simulink model "Communication2_2018a"  (R2018a)
settings: Solver=VariableStepAuto  StartTime=0.0  StopTime=0.6  RelTol=1e-3
settings Model: Creator=86188  LastModifiedBy=bzhan

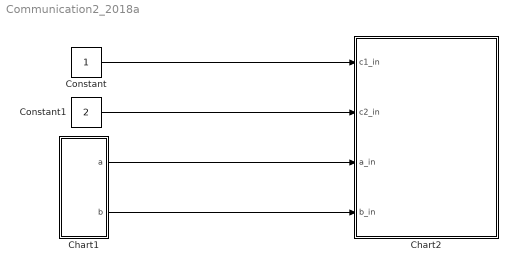
== system Communication2_2018a ==
  Chart1 : Stateflow chart  TreatAsAtomicUnit=on
  Chart2 : Stateflow chart  TreatAsAtomicUnit=on
  Constant : Constant
  Constant1 : Constant  Value=2
  wires:
  Constant1/1 -> Chart2/2(c2_in)
  Constant/1 -> Chart2/1(c1_in)
  Chart1/1(a) -> Chart2/3(a_in)
  Chart1/2(b) -> Chart2/4(b_in)

== stateflow chart Communication2_2018a/Chart2 ==
  settings: updateMethod=DISCRETE  sampleTime=0.1
  state A1
    en: g("en_A1");
    du: f();
  (default) -> A1
  data: s function_input; c1_in input; c2_in input; y local =0; a_in input; b_in input
  function f:
    | function f()
    |   fprintf("%.0f %.0f %.0f %.0f\n", c1_in, c2_in, a_in, b_in);
  function g(s):
    | function g(s)
    |   fprintf(s+"\n");

== stateflow chart Communication2_2018a/Chart1 ==
  settings: updateMethod=DISCRETE  sampleTime=0.1
  state A
    en: f("en_A")
  state B
    en:
    f("en_B")
  (default) -> A : {a=1;b=1;}
  A -> B : {a=a+1;}
  B -> A : {b=b+1;}
  data: s function_input; i local; a output; b output
  function f(s):
    | function f(s)
    |   fprintf(s+"\n");
